simulink model "MyPTControlOSM_RTW"  (Simulink 7.5)
settings: Solver=ode1  SolverMode=SingleTasking  StartTime=0.0  StopTime=inf  FixedStep=0.0002  RelTol=1e-3
PreLoadFcn:
  | vehicle = 'Car'; if ~length(which('cmcmd')), cmenv; end
  | MyPTControlOSM_RTW_bus
InitFcn:
  | vehicle = 'Car'; if ~length(which('cmcmd')), cmenv; end
  | MyPTControlOSM_RTW_bus
undefined symbols (not defined in the file or in its folder): OperationState, OSMFunc, rv, State
libraries: simulink x14
(part 2 of 2)

== system MyPTControlOSM_RTW/MyPTControlOSM/PowerOn/SkipStart function exist? ==
  Bus In : Inport  OutDataType=sfix(16)  OutScaling=2^0
  Input : Inport  Port=2  OutDataType=sfix(16)  OutScaling=2^0
  State 4 SkipStart function exist? : ActionPort  ActionType=case
  Bus Creator : BusCreator
  Bus Selector1 : BusSelector  OutputSignals=OSMFunc
  Bus Selector2 : BusSelector  OutputSignals=rv,OperationState
  Bus Selector3 : BusSelector  OutputSignals=Func_used.OSMFunc_SkipStart
  Constant2 : Constant  Value=5  OutDataType=sfix(16)  OutScaling=2^0
  Constant3 : Constant  Value=6  OutDataType=sfix(16)  OutScaling=2^0
  Demux : Demux  Outputs=2
  Mux : Mux  Inputs=2
  Mux1 : Mux  Inputs=2
  OSMFunc_SkipStart : Constant  Value=6  OutDataType=sfix(16)  OutScaling=2^0
  Signal Conversion : SignalConversion  ConversionOutput=Bus copy
  Switch1 : Switch  Criteria=u2 ~= 0  OutDataType=sfix(16)  OutScaling=2^0
  Bus Out : Outport  OutDataType=sfix(16)  OutScaling=2^0
  wires:
  Bus In/1 -> Bus Selector1/1, Bus Selector2/1
  Bus Creator/1 -> Signal Conversion/1
  Input/1 -> Bus Selector3/1
  Switch1/1 -> Demux/1
  Mux/1 -> Switch1/3
  Bus Selector1/1 -> Mux/1  "<OSMFunc>"
  Constant3/1 -> Mux/2  "State"
  Signal Conversion/1 -> Bus Out/1
  Bus Selector2/2 -> Bus Creator/2  "<OperationState>"
  Demux/1 -> Bus Creator/3  "OSMFunc"
  Demux/2 -> Bus Creator/4  "State"
  Bus Selector3/1 -> Switch1/2  "<OSMFunc_SkipStart>"
  Bus Selector2/1 -> Bus Creator/1  "<rv>"
  Constant2/1 -> Mux1/2  "State"
  OSMFunc_SkipStart/1 -> Mux1/1
  Mux1/1 -> Switch1/1

== system MyPTControlOSM_RTW/MyPTControlOSM/PowerOn/SkipStart reached -> PowerOn function exist? ==
  Bus In : Inport  OutDataType=sfix(16)  OutScaling=2^0
  Input : Inport  Port=2  OutDataType=sfix(16)  OutScaling=2^0
  "State 6 SkipStart reached -> PowerOn function exist?" : ActionPort  ActionType=case
  Bus Creator : BusCreator
  Bus Selector1 : BusSelector  OutputSignals=OSMFunc
  Bus Selector2 : BusSelector  OutputSignals=rv,OperationState
  Bus Selector3 : BusSelector  OutputSignals=Func_used.OSMFunc_PowerOn
  Constant2 : Constant  Value=7  OutDataType=sfix(16)  OutScaling=2^0
  Constant3 : Constant  Value=8  OutDataType=sfix(16)  OutScaling=2^0
  Demux : Demux  Outputs=2
  Mux : Mux  Inputs=2
  Mux1 : Mux  Inputs=2
  OSMFunc_PowerOn : Constant  Value=4  OutDataType=sfix(16)  OutScaling=2^0
  Signal Conversion1 : SignalConversion  ConversionOutput=Bus copy
  Switch1 : Switch  Criteria=u2 ~= 0  OutDataType=sfix(16)  OutScaling=2^0
  Bus Out : Outport  OutDataType=sfix(16)  OutScaling=2^0
  wires:
  Bus In/1 -> Bus Selector1/1, Bus Selector2/1
  Bus Creator/1 -> Signal Conversion1/1
  Input/1 -> Bus Selector3/1
  Switch1/1 -> Demux/1
  Mux/1 -> Switch1/3
  Bus Selector1/1 -> Mux/1  "<OSMFunc>"
  Constant3/1 -> Mux/2  "State"
  Signal Conversion1/1 -> Bus Out/1
  Bus Selector2/2 -> Bus Creator/2  "<OperationState>"
  Demux/1 -> Bus Creator/3  "OSMFunc"
  Demux/2 -> Bus Creator/4  "State"
  Bus Selector3/1 -> Switch1/2  "<OSMFunc_PowerOn>"
  Bus Selector2/1 -> Bus Creator/1  "<rv>"
  Constant2/1 -> Mux1/2  "State"
  OSMFunc_PowerOn/1 -> Mux1/1
  Mux1/1 -> Switch1/1

== system MyPTControlOSM_RTW/MyPTControlOSM/PowerOn/Start function exist? ==
  Bus In : Inport  OutDataType=sfix(16)  OutScaling=2^0
  Input : Inport  Port=2  OutDataType=sfix(16)  OutScaling=2^0
  State 1 Start function exist? : ActionPort  ActionType=case
  Bus Creator : BusCreator
  Bus Selector1 : BusSelector  OutputSignals=OSMFunc
  Bus Selector2 : BusSelector  OutputSignals=rv,OperationState
  Bus Selector3 : BusSelector  OutputSignals=Func_used.OSMFunc_SkipStart
  Constant2 : Constant  Value=2  OutDataType=sfix(16)  OutScaling=2^0
  Constant3 : Constant  Value=3  OutDataType=sfix(16)  OutScaling=2^0
  Demux : Demux  Outputs=2
  Mux : Mux  Inputs=2
  Mux1 : Mux  Inputs=2
  OSMFunc_Start : Constant  Value=5  OutDataType=sfix(16)  OutScaling=2^0
  Signal Conversion1 : SignalConversion  ConversionOutput=Bus copy
  Switch1 : Switch  Criteria=u2 ~= 0  OutDataType=sfix(16)  OutScaling=2^0
  Bus Out : Outport  OutDataType=sfix(16)  OutScaling=2^0
  wires:
  Bus In/1 -> Bus Selector1/1, Bus Selector2/1
  Bus Creator/1 -> Signal Conversion1/1
  Input/1 -> Bus Selector3/1
  Switch1/1 -> Demux/1
  Mux/1 -> Switch1/3
  Bus Selector1/1 -> Mux/1  "<OSMFunc>"
  Constant3/1 -> Mux/2  "State"
  Signal Conversion1/1 -> Bus Out/1
  Bus Selector2/2 -> Bus Creator/2  "<OperationState>"
  Demux/1 -> Bus Creator/3  "OSMFunc"
  Demux/2 -> Bus Creator/4  "State"
  Bus Selector3/1 -> Switch1/2  "<OSMFunc_SkipStart>"
  Constant2/1 -> Mux1/2  "State"
  OSMFunc_Start/1 -> Mux1/1
  Mux1/1 -> Switch1/1
  Bus Selector2/1 -> Bus Creator/1  "<rv>"

== system MyPTControlOSM_RTW/MyPTControlOSM/PowerOn/Wait for PowerOff is ready ==
  Bus In : Inport  OutDataType=sfix(16)  OutScaling=2^0
  Input : Inport  Port=2  OutDataType=sfix(16)  OutScaling=2^0
  State 10 Wait for PowerOff is ready : ActionPort  ActionType=case
  Bus Assignment : BusAssignment  AssignedSignals=State
  Bus Selector : BusSelector  OutputSignals=FuncReturn
  Constant : Constant  Value=11  OutDataType=sfix(16)  OutScaling=2^0
  Constant1 : Constant  Value=10  OutDataType=sfix(16)  OutScaling=2^0
  Signal Conversion : SignalConversion  ConversionOutput=Bus copy
  Switch : Switch  Criteria=u2 ~= 0  OutDataType=sfix(16)  OutScaling=2^0
  Bus Out : Outport  OutDataType=sfix(16)  OutScaling=2^0
  wires:
  Signal Conversion/1 -> Bus Out/1
  Bus Assignment/1 -> Signal Conversion/1
  Bus In/1 -> Bus Assignment/1
  Input/1 -> Bus Selector/1
  Bus Selector/1 -> Switch/2  "<FuncReturn>"
  Constant/1 -> Switch/1
  Constant1/1 -> Switch/3
  Switch/1 -> Bus Assignment/2

== system MyPTControlOSM_RTW/MyPTControlOSM/PowerOn/Wait for PowerOn is ready ==
  Bus In : Inport  OutDataType=sfix(16)  OutScaling=2^0
  Input : Inport  Port=2  OutDataType=sfix(16)  OutScaling=2^0
  State 7 Wait for PowerOn is ready : ActionPort  ActionType=case
  Bus Assignment : BusAssignment  AssignedSignals=State
  Bus Selector : BusSelector  OutputSignals=FuncReturn
  Constant : Constant  Value=8  OutDataType=sfix(16)  OutScaling=2^0
  Constant1 : Constant  Value=7  OutDataType=sfix(16)  OutScaling=2^0
  Signal Conversion : SignalConversion  ConversionOutput=Bus copy
  Switch : Switch  Criteria=u2 ~= 0  OutDataType=sfix(16)  OutScaling=2^0
  Bus Out : Outport  OutDataType=sfix(16)  OutScaling=2^0
  wires:
  Signal Conversion/1 -> Bus Out/1
  Bus Assignment/1 -> Signal Conversion/1
  Bus In/1 -> Bus Assignment/1
  Input/1 -> Bus Selector/1
  Bus Selector/1 -> Switch/2  "<FuncReturn>"
  Constant/1 -> Switch/1
  Constant1/1 -> Switch/3
  Switch/1 -> Bus Assignment/2

== system MyPTControlOSM_RTW/MyPTControlOSM/PowerOn/Wait for SkipStart is ready ==
  Bus In : Inport  OutDataType=sfix(16)  OutScaling=2^0
  Input : Inport  Port=2  OutDataType=sfix(16)  OutScaling=2^0
  State 5 Wait for SkipStart is ready : ActionPort  ActionType=case
  Bus Assignment : BusAssignment  AssignedSignals=State
  Bus Selector : BusSelector  OutputSignals=FuncReturn
  Constant : Constant  Value=6  OutDataType=sfix(16)  OutScaling=2^0
  Constant1 : Constant  Value=5  OutDataType=sfix(16)  OutScaling=2^0
  Signal Conversion : SignalConversion  ConversionOutput=Bus copy
  Switch : Switch  Criteria=u2 ~= 0  OutDataType=sfix(16)  OutScaling=2^0
  Bus Out : Outport  OutDataType=sfix(16)  OutScaling=2^0
  wires:
  Signal Conversion/1 -> Bus Out/1
  Bus Assignment/1 -> Signal Conversion/1
  Bus In/1 -> Bus Assignment/1
  Input/1 -> Bus Selector/1
  Bus Selector/1 -> Switch/2  "<FuncReturn>"
  Constant/1 -> Switch/1
  Constant1/1 -> Switch/3
  Switch/1 -> Bus Assignment/2

== system MyPTControlOSM_RTW/MyPTControlOSM/PowerOn/Wait for Start is ready ==
  Bus In : Inport  OutDataType=sfix(16)  OutScaling=2^0
  Input : Inport  Port=2  OutDataType=sfix(16)  OutScaling=2^0
  State 2 Wait for Start is ready : ActionPort  ActionType=case
  !=KeyPos_KeyIn_Starter : simulink/Logic and Bit Operations/Compare To Constant  SystemSampleTime=-1  relop=~=  const=4  LogicOutDataTypeMode=uint8  ZeroCross=off
  Bus Assignment : BusAssignment  AssignedSignals=State
  Bus Selector : BusSelector  OutputSignals=FuncReturn
  Bus Selector1 : BusSelector  OutputSignals=Key
  Constant : Constant  Value=4  OutDataType=sfix(16)  OutScaling=2^0
  Constant1 : Constant  Value=2  OutDataType=sfix(16)  OutScaling=2^0
  Constant2 : Constant  Value=3  OutDataType=sfix(16)  OutScaling=2^0
  Input Copy : InportShadow  Port=2  OutDataType=sfix(16)  OutScaling=2^0
  Signal Conversion : SignalConversion  ConversionOutput=Bus copy
  Skip Start if Key ist not Starter : Switch  Criteria=u2 ~= 0  OutDataType=sfix(16)  OutScaling=2^0
  Switch : Switch  Criteria=u2 ~= 0  OutDataType=sfix(16)  OutScaling=2^0
  Bus Out : Outport  OutDataType=sfix(16)  OutScaling=2^0
  wires:
  Bus Assignment/1 -> Signal Conversion/1
  Signal Conversion/1 -> Bus Out/1
  Bus In/1 -> Bus Assignment/1
  Skip Start if Key ist not Starter/1 -> Switch/3
  Switch/1 -> Bus Assignment/2
  !=KeyPos_KeyIn_Starter/1 -> Skip Start if Key ist not Starter/2
  Constant/1 -> Skip Start if Key ist not Starter/1
  Constant1/1 -> Skip Start if Key ist not Starter/3
  Input Copy/1 -> Bus Selector/1
  Input/1 -> Bus Selector1/1
  Bus Selector1/1 -> !=KeyPos_KeyIn_Starter/1  "<Key>"
  Bus Selector/1 -> Switch/2  "<FuncReturn>"
  Constant2/1 -> Switch/1

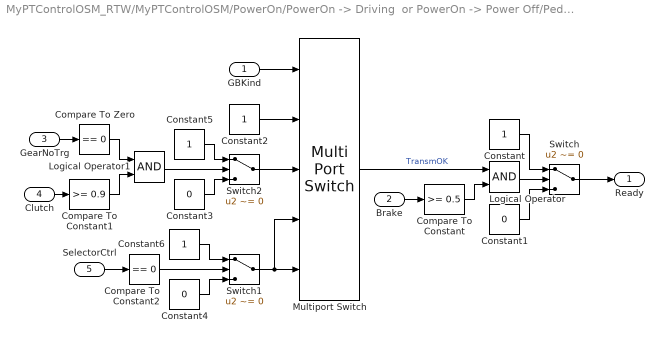
== system MyPTControlOSM_RTW/MyPTControlOSM/PowerOn/PowerOn -> Driving  or PowerOn -> Power Off/PedalsReady2Start ==
  GBKind : Inport  OutDataType=sfix(16)  OutScaling=2^0
  Brake : Inport  Port=2  OutDataType=sfix(16)  OutScaling=2^0
  GearNoTrg : Inport  Port=3  OutDataType=sfix(16)  OutScaling=2^0
  Clutch : Inport  Port=4  OutDataType=sfix(16)  OutScaling=2^0
  SelectorCtrl : Inport  Port=5  OutDataType=sfix(16)  OutScaling=2^0
  Compare To Constant : simulink/Logic and Bit Operations/Compare To Constant  SystemSampleTime=-1  relop=>=  const=0.5  LogicOutDataTypeMode=uint8  ZeroCross=off
  Compare To Constant1 : simulink/Logic and Bit Operations/Compare To Constant  SystemSampleTime=-1  relop=>=  const=0.9  LogicOutDataTypeMode=uint8  ZeroCross=off
  Compare To Constant2 : simulink/Logic and Bit Operations/Compare To Constant  SystemSampleTime=-1  relop===  const=0  LogicOutDataTypeMode=uint8  ZeroCross=off
  Compare To Zero : simulink/Logic and Bit Operations/Compare To Zero  SystemSampleTime=-1  relop===  LogicOutDataTypeMode=uint8  ZeroCross=off
  Constant{,2,5..6} (4 alike) : Constant  OutDataType=sfix(16)  OutScaling=2^0
  Constant1 : Constant  Value=0  OutDataType=sfix(16)  OutScaling=2^0
  Constant3 : Constant  Value=0  OutDataType=sfix(16)  OutScaling=2^0
  Constant4 : Constant  Value=0  OutDataType=sfix(16)  OutScaling=2^0
  Logical Operator : Logic  AllPortsSameDT=off  OutDataTypeMode=boolean  OutDataTypeStr=boolean
  Logical Operator1 : Logic  AllPortsSameDT=off  OutDataTypeMode=boolean  OutDataTypeStr=boolean
  Multiport Switch : MultiPortSwitch  DataPortOrder=Zero-based contiguous  Inputs=4  zeroidx=on  OutDataType=sfix(16)  OutScaling=2^0
  Switch : Switch  Criteria=u2 ~= 0  OutDataType=sfix(16)  OutScaling=2^0
  Switch1 : Switch  Criteria=u2 ~= 0  OutDataType=sfix(16)  OutScaling=2^0
  Switch2 : Switch  Criteria=u2 ~= 0  OutDataType=sfix(16)  OutScaling=2^0
  Ready : Outport  OutDataType=sfix(16)  OutScaling=2^0
  wires:
  GBKind/1 -> Multiport Switch/1
  Multiport Switch/1 -> Logical Operator/1  "TransmOK"
  Brake/1 -> Compare To Constant/1
  Compare To Constant/1 -> Logical Operator/2
  Switch/1 -> Ready/1
  Logical Operator/1 -> Switch/2
  Constant1/1 -> Switch/3
  Constant/1 -> Switch/1
  Constant2/1 -> Multiport Switch/2
  Switch1/1 -> Multiport Switch/5, Multiport Switch/4
  Switch2/1 -> Multiport Switch/3
  Constant3/1 -> Switch2/3
  Constant4/1 -> Switch1/3
  Constant5/1 -> Switch2/1
  Constant6/1 -> Switch1/1
  Logical Operator1/1 -> Switch2/2
  Clutch/1 -> Compare To Constant1/1
  GearNoTrg/1 -> Compare To Zero/1
  Compare To Zero/1 -> Logical Operator1/1
  Compare To Constant1/1 -> Logical Operator1/2
  SelectorCtrl/1 -> Compare To Constant2/1
  Compare To Constant2/1 -> Switch1/2
